simulink model "Q2a_Simulink"  (R2021a)
settings: Solver=VariableStepAuto  StartTime=0.0  StopTime=2/60  RelTol=1e-3
libraries: fl_lib x10, nesl_utility x7, spsFourierLib x2, ee_lib x2
settings Model: Creator=bemen  LastModifiedBy=bemen

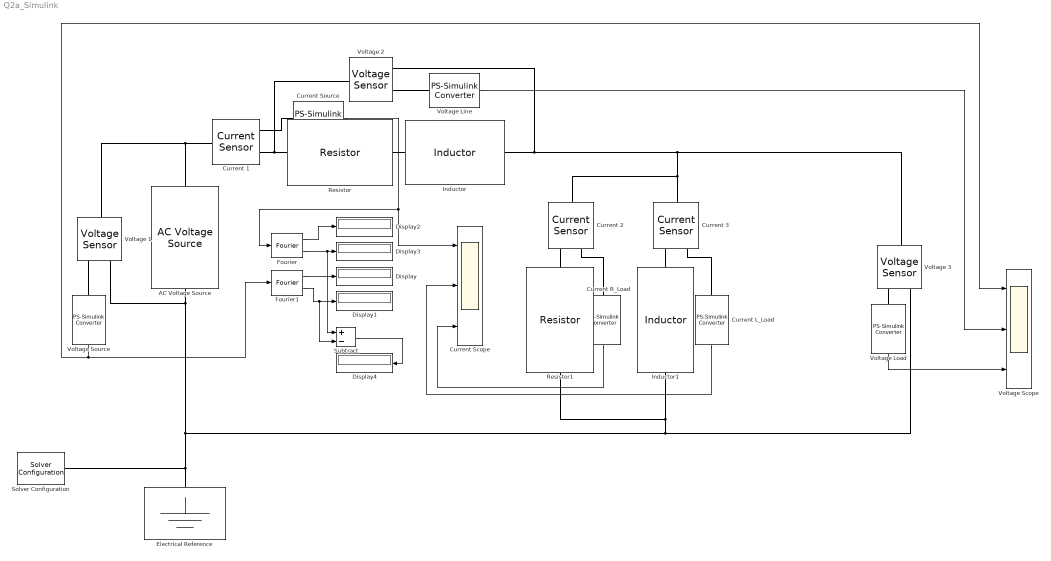
== system Q2a_Simulink ==
  AC Voltage Source : fl_lib/Electrical/Electrical Sources/AC Voltage Source  amp=120 V  shift=0 deg  frequency=60 Hz  omega=0 rad/s
  Current 1 : fl_lib/Electrical/Electrical Sensors/Current Sensor
  Current 2 : fl_lib/Electrical/Electrical Sensors/Current Sensor
  Current 3 : fl_lib/Electrical/Electrical Sensors/Current Sensor
  Current L_Load : nesl_utility/PS-Simulink Converter  PhysicalDomain=network_engine_domain  SubClassName=ps_output  LeftPortType=input  RightPortType=output  PseudoPeriodic=off  Frequencies=[]  Unit=inherit  AffineConversion=off
      settings: SourceProductBaseCode=PW,SS
  Current R_Load : nesl_utility/PS-Simulink Converter  PhysicalDomain=network_engine_domain  SubClassName=ps_output  LeftPortType=input  RightPortType=output  PseudoPeriodic=off  Frequencies=[]  Unit=inherit  AffineConversion=off
      settings: SourceProductBaseCode=PW,SS
  Current Scope : Scope  NumInputPorts=3
  Current Source : nesl_utility/PS-Simulink Converter  PhysicalDomain=network_engine_domain  SubClassName=ps_output  LeftPortType=input  RightPortType=output  PseudoPeriodic=off  Frequencies=[]  Unit=inherit  AffineConversion=off
      settings: SourceProductBaseCode=PW,SS
  Display{,1..4} (5 alike) : Display
  Electrical Reference : fl_lib/Electrical/Electrical Elements/Electrical Reference
  Fourier : spsFourierLib/Fourier  Freq=60  n=1  InInit=[0, 0]  Ts=0
      settings: SourceProductBaseCode=PS
  Fourier1 : spsFourierLib/Fourier  Freq=60  n=1  InInit=[0, 0]  Ts=0
      settings: SourceProductBaseCode=PS
  Inductor : fl_lib/Electrical/Electrical Elements/Inductor  l=2.65 mH  r=0 Ohm  g=1e-9 1/Ohm  i_specify=off  i_priority=None  i=0 A  i_nominal_specify=off  i_nominal_unit=A  i_nominal_value=1  v_specify=off  v_priority=None  v=0 V  v_nominal_specify=off  v_nominal_unit=V  v_nominal_value=1  i_L_specify=off  i_L_priority=High  i_L=0 A  i_L_nominal_specify=off  i_L_nominal_unit=A  i_L_nominal_value=1
  Inductor1 : fl_lib/Electrical/Electrical Elements/Inductor  l=26.5 mH  r=0 Ohm  g=1e-9 1/Ohm  i_specify=off  i_priority=None  i=0 A  i_nominal_specify=off  i_nominal_unit=A  i_nominal_value=1  v_specify=off  v_priority=None  v=0 V  v_nominal_specify=off  v_nominal_unit=V  v_nominal_value=1  i_L_specify=off  i_L_priority=High  i_L=0 A  i_L_nominal_specify=off  i_L_nominal_unit=A  i_L_nominal_value=1
  Resistor : ee_lib/Passive/Resistor  R=1 Ohm  R_tol=5  enable_R_tol=0  tol_distribution=1  nSigma=4  enable_operating_limits=0  operating_limit_action=2  max_working_voltage=100 V  power_rating=1 W  enable_faults=0  fault_action=1  R_faulted=inf Ohm  enable_temporal_fault=0  t_fault=1 s  enable_behavioral_fault=0  max_permissible_current=1 A  t_fail_on_current=1 s  noise_mode=0  sample_time=1e-3 s  repeatability=1  auto_seed=3499211588  user_seed=0  Tdevice=25 degC  alpha=3.93e-3 1/K  Tmeas=25 degC  thermal_mass=100 J/K  power_derating_T1=70 degC  power_derating_T2=155 degC  operating_temperature_range_vec=[-50, 150] degC  temperature_specify=off  temperature_priority=High  temperature=298.15 K  temperature_nominal_specify=off  temperature_nominal_unit=K  temperature_nominal_value=1
  Resistor1 : ee_lib/Passive/Resistor  R=10 Ohm  R_tol=5  enable_R_tol=0  tol_distribution=1  nSigma=4  enable_operating_limits=0  operating_limit_action=2  max_working_voltage=100 V  power_rating=1 W  enable_faults=0  fault_action=1  R_faulted=inf Ohm  enable_temporal_fault=0  t_fault=1 s  enable_behavioral_fault=0  max_permissible_current=1 A  t_fail_on_current=1 s  noise_mode=0  sample_time=1e-3 s  repeatability=1  auto_seed=3890346746  user_seed=0  Tdevice=25 degC  alpha=3.93e-3 1/K  Tmeas=25 degC  thermal_mass=100 J/K  power_derating_T1=70 degC  power_derating_T2=155 degC  operating_temperature_range_vec=[-50, 150] degC  temperature_specify=off  temperature_priority=High  temperature=298.15 K  temperature_nominal_specify=off  temperature_nominal_unit=K  temperature_nominal_value=1
  Solver Configuration : nesl_utility/Solver Configuration  PhysicalDomain=network_engine_domain  SubClassName=solver  LeftPortType=input  RightPortType=generic  Tones=[]  Harmonics=[]  SimulateNoise=off  Profile=off  UseLocalSampling=off  EnableSwitchedLinearOptims=on  FrequencyDomain=off  UseCCode=off  RelTol=0.001  AbsTol=1e-06  MinStep=1e-09  ToWorkspace=off  RevertToSquareIcSolve=off  NumHomotopyIterations=100  PhasorMode=off  PhasorModeNumHarmonics=1  DoDC=on  ResidualTolerance=1e-10  UseLocalSolver=off  LocalSolverChoice=NE_BACKWARD_EULER_ADVANCER  LocalSolverSampleTime=0.001  DoFixedCost=off  MaxNonlinIter=3  MaxModeIter=2  ComputeImpulses=off  ImpulseIterations=2  LinearAlgebra=auto  EquationFormulation=NE_TIME_EF  DelaysMemoryBudget=1024  AutomaticFiltering=on  FilteringTimeConstant=0.0001  PartitionStorageMethod=AS_NEEDED  PartitionMemoryBudget=1024  PartitionMethod=ROBUST
      settings: SourceProductBaseCode=PW,SS
  Subtract : Sum  Inputs=+-
  Voltage 1 : fl_lib/Electrical/Electrical Sensors/Voltage Sensor
  Voltage 2 : fl_lib/Electrical/Electrical Sensors/Voltage Sensor
  Voltage 3 : fl_lib/Electrical/Electrical Sensors/Voltage Sensor
  Voltage Line : nesl_utility/PS-Simulink Converter  PhysicalDomain=network_engine_domain  SubClassName=ps_output  LeftPortType=input  RightPortType=output  PseudoPeriodic=off  Frequencies=[]  Unit=inherit  AffineConversion=off
      settings: SourceProductBaseCode=PW,SS
  Voltage Load : nesl_utility/PS-Simulink Converter  PhysicalDomain=network_engine_domain  SubClassName=ps_output  LeftPortType=input  RightPortType=output  PseudoPeriodic=off  Frequencies=[]  Unit=inherit  AffineConversion=off
      settings: SourceProductBaseCode=PW,SS
  Voltage Scope : Scope  NumInputPorts=3
  Voltage Source : nesl_utility/PS-Simulink Converter  PhysicalDomain=network_engine_domain  SubClassName=ps_output  LeftPortType=input  RightPortType=output  PseudoPeriodic=off  Frequencies=[]  Unit=inherit  AffineConversion=off
      settings: SourceProductBaseCode=PW,SS
  wires:
  Voltage Source/1 -> Voltage Scope/1, Fourier1/1
  Voltage Line/1 -> Voltage Scope/2
  Voltage Load/1 -> Voltage Scope/3
  Current R_Load/1 -> Current Scope/3
  Current L_Load/1 -> Current Scope/2
  Current Source/1 -> Fourier/1, Current Scope/1
  Fourier/2 -> Subtract/1, Display3/1
  Fourier/1 -> Display2/1
  Fourier1/1 -> Display/1
  Fourier1/2 -> Subtract/2, Display1/1
  Subtract/1 -> Display4/1
  connections:
  Electrical Reference/LConn1 -- Voltage 3/RConn2 -- Resistor1/RConn1 -- Inductor1/RConn1 -- Voltage 1/RConn2 -- AC Voltage Source/RConn1 -- Solver Configuration/RConn1
  Resistor/RConn1 -- Inductor/LConn1
  Resistor1/LConn1 -- Current 2/RConn2
  Inductor1/LConn1 -- Current 3/RConn2
  AC Voltage Source/LConn1 -- Voltage 1/LConn1 -- Current 1/LConn1
  Current 1/RConn2 -- Voltage 2/LConn1 -- Resistor/LConn1
  Inductor/RConn1 -- Voltage 3/LConn1 -- Current 2/LConn1 -- Current 3/LConn1 -- Voltage 2/RConn2
  Voltage Source/LConn1 -- Voltage 1/RConn1
  Voltage 2/RConn1 -- Voltage Line/LConn1
  Current R_Load/LConn1 -- Current 2/RConn1
  Current 3/RConn1 -- Current L_Load/LConn1
  Current 1/RConn1 -- Current Source/LConn1
  Voltage Load/LConn1 -- Voltage 3/RConn1
